simulink subsystem "ControlProporcional"  (R2021b)
settings: Solver=VariableStepAuto  StartTime=0.0  StopTime=10.0  RelTol=1e-3
settings Model: Creator=yo  LastModifiedBy=yo

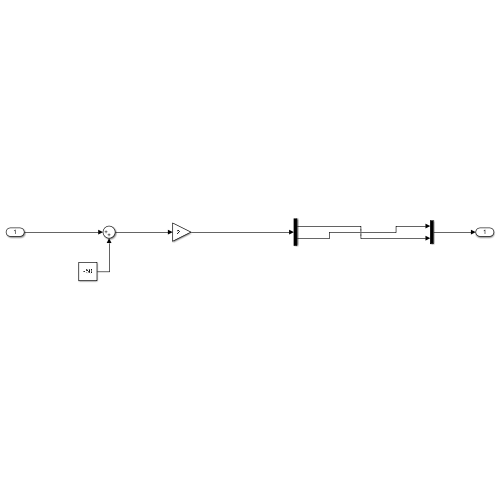
[thumbnail: Simulink's stored preview of the top-level diagram]
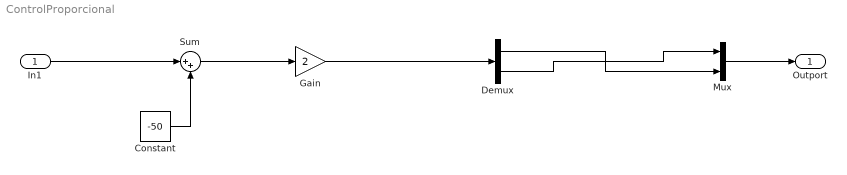
== system ControlProporcional ==
  In1 : Inport
  Constant : Constant  Value=-50
  Demux : Demux  Outputs=2
  Gain : Gain  Gain=2
  Mux : Mux  Inputs=2
  Sum : Sum  Inputs=|++
  Outport : Outport
  wires:
  Demux/2 -> Mux/1
  In1/1 -> Sum/1
  Demux/1 -> Mux/2
  Mux/1 -> Outport/1
  Constant/1 -> Sum/2
  Gain/1 -> Demux/1
  Sum/1 -> Gain/1
